simulink model "Practica1MSF "  (R2025b)
settings: Solver=VariableStepAuto  StartTime=0.0  StopTime=10  MaxStep=1E-3  RelTol=1e-3
libraries: slpidlib x1, simulink x1
settings DataIOCC: ReturnWorkspaceOutputs=off  TimeSaveName=t
settings DebuggingCC: AlgebraicLoopMsg=none  ArtificialAlgebraicLoopMsg=none  MaxConsecutiveZCsMsg=none

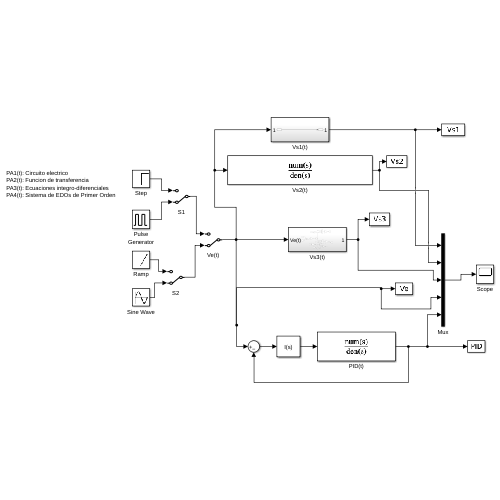
[thumbnail: Simulink's stored preview of the top-level diagram]
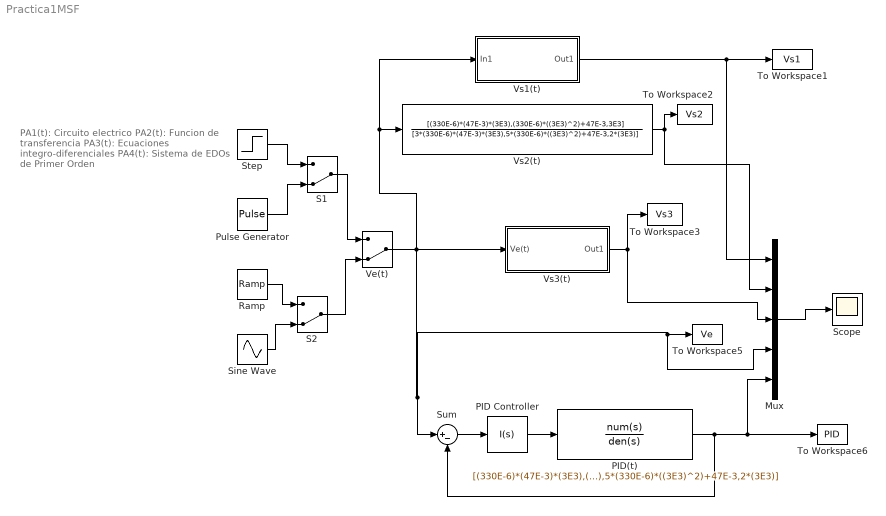
== system Practica1MSF  ==
  note: PA1(t): Circuito electrico
      | PA2(t): Funcion de transferencia
      | PA3(t): Ecuaciones integro-diferenciales
      | PA4(t): Sistema de EDOs de Primer Orden
  Mux : Mux  Inputs=5
  PID Controller : slpidlib/PID Controller  Controller=I  Form=Parallel  TimeDomain=Continuous-time  UseExternalTs=off  SampleTime=-1  IntegratorMethod=Forward Euler  FilterMethod=Forward Euler  ControllerParametersSource=internal  P=1  I=1961.8958  UseKiTs=off  D=1  UseExternalDerivativeSource=off  N=1  UseFilter=on  TunerSelectOption=Transfer Function Based (PID Tuner App)  InitialConditionSource=internal  InitialConditionForIntegrator=0  InitialConditionForFilter=0  DifferentiatorICPrevScaledInput=0  ExternalReset=none  TrackingMode=off  Kt=1  LimitOutput=off  SatLimitsSource=internal  UpperSaturationLimit=inf  LowerSaturationLimit=-inf  LinearizeAsGain=on  AntiWindupMode=none  Kb=1  LimitIntegrator=off  UpperIntegratorSaturationLimit=inf  LowerIntegratorSaturationLimit=-inf  POutMin=[]  POutMax=[]  IOutMin=[]  IOutMax=[]  DOutMin=[]  DOutMax=[]  NOutMin=[]  NOutMax=[]  SumOutMin=[]  SumOutMax=[]  SaturationOutMin=[]  SaturationOutMax=[]  PParamMin=[]  PParamMax=[]  IParamMin=[]  IParamMax=[]  DParamMin=[]  DParamMax=[]  NParamMin=[]  NParamMax=[]  KbParamMin=[]  KbParamMax=[]  KtParamMin=[]  KtParamMax=[]  KbOutMin=[]  KbOutMax=[]  KtOutMin=[]  KtOutMax=[]  IntegratorOutMin=[]  IntegratorOutMax=[]  FilterOutMin=[]  FilterOutMax=[]  SumI1OutMin=[]  SumI1OutMax=[]  SumI2OutMin=[]  SumI2OutMax=[]  SumI3OutMin=[]  SumI3OutMax=[]  SumI4OutMin=[]  SumI4OutMax=[]  SumDOutMin=[]  SumDOutMax=[]  DifferentiatorOutMin=[]  DifferentiatorOutMax=[]  FilterDiffOutCoefMin=[]  FilterDiffOutCoefMax=[]  ReciprocalOutMin=[]  ReciprocalOutMax=[]  SumDenOutMin=[]  SumDenOutMax=[]  SumNumOutMin=[]  SumNumOutMax=[]  DivideOutMin=[]  DivideOutMax=[]  UdiffTsProdOutMin=[]  UdiffTsProdOutMax=[]  NTsProdOutMin=[]  NTsProdOutMax=[]  UintegralTsProdOutMin=[]  UintegralTsProdOutMax=[]  UngainTsProdOutMin=[]  UngainTsProdOutMax=[]  ClampingZeroOutDataTypeStr=Inherit: Inherit via back propagation  ClampingZeroOutMin=[]  ClampingZeroOutMax=[]  FilterDenConstantOutDataTypeStr=Inherit: Inherit via back propagation  FilterDenConstantOutMin=[]  FilterDenConstantOutMax=[]  PCopyOutDataTypeStr=Inherit: Inherit via back propagation  PCopyOutMin=[]  PCopyOutMax=[]  NCopyOutDataTypeStr=Inherit: Inherit via back propagation  NCopyOutMin=[]  NCopyOutMax=[]  IntegratorContinuousStateAttributes=''  IntegratorStateMustResolveToSignalObject=off  IntegratorRTWStateStorageClass=Auto  FilterContinuousStateAttributes=''  FilterStateMustResolveToSignalObject=off  FilterRTWStateStorageClass=Auto  ParallelPVariant=Disabled  IdealPVariant=Disabled  IVariant=InternalParameters  DVariant=Disabled  IntegratorVariant=Continuous  SatVariant=Disabled  AWVariant=Passthrough  PCopyVariant=Disabled  TRVariant=Disabled  FdbkBlocksVariant=Forward  IdealPFdbkVariant=Disabled  SatFdbkVariant=Disabled  DerivativeFilterVariant=Disabled  NVariant=Disabled  NCopyVariant=Disabled_SignalSpec  FilterICVariant=Disabled  IntegratorICVariant=InternalICs  ExternalResetVariant=Disabled  TRSumVariant=Passthrough  SumFdbkVariant=Disabled  SumVariant=Passthrough_I  TsampFilterVariant=InternalTs  TsampNgainVariant=Passthrough  TsampIntegralVariant=Disabled_SignalSpec  ExternalSaturationOutDataTypeStr=Inherit: Same as second input  DerivativeSourceVariant=Disabled  PreIntVariant=InternalPreInt
  PID(t) : TransferFcn  Numerator=[(330E-6)*(47E-3)*(3E3),(330E-6)*((3E3)^2)+47E-3,3E3]  Denominator=[3*(330E-6)*(47E-3)*(3E3),5*(330E-6)*((3E3)^2)+47E-3,2*(3E3)]
  Pulse Generator : DiscretePulseGenerator  PulseType=Time based  Period=10  PulseWidth=10  PhaseDelay=1
  Ramp : simulink/Sources/Ramp  slope=1/10  start=0  InitialOutput=0
  S1 : ManualSwitch  CurrentSetting=0
  S2 : ManualSwitch  CurrentSetting=0
  Scope : Scope
      settings: ActiveDisplayYMinimum=-0.12518759179665592  ActiveDisplayYMaximum=1.1266883261699037
  Sine Wave : Sin  Frequency=pi/2  SampleTime=0
  Step : Step  Time=0  Before=1  SampleTime=0
  Sum : Sum  Inputs=|+-
  To Workspace1 : ToWorkspace  VariableName=Vs1  SampleTime=-1
  To Workspace2 : ToWorkspace  VariableName=Vs2  SampleTime=-1
  To Workspace3 : ToWorkspace  VariableName=Vs3  SampleTime=-1
  To Workspace5 : ToWorkspace  VariableName=Ve  SampleTime=-1
  To Workspace6 : ToWorkspace  VariableName=PID  SampleTime=-1
  Ve(t) : ManualSwitch  CurrentSetting=0
  Vs1(t) : Subsystem
  Vs2(t) : TransferFcn  Numerator=[(330E-6)*(47E-3)*(3E3),(330E-6)*((3E3)^2)+47E-3,3E3]  Denominator=[3*(330E-6)*(47E-3)*(3E3),5*(330E-6)*((3E3)^2)+47E-3,2*(3E3)]
  Vs3(t) : Subsystem
  wires:
  Step/1 -> S1/1
  Pulse Generator/1 -> S1/2
  Ramp/1 -> S2/1
  Sine Wave/1 -> S2/2
  S1/1 -> Ve(t)/1
  S2/1 -> Ve(t)/2
  Vs2(t)/1 -> To Workspace2/1, Mux/2
  Ve(t)/1 -> Vs3(t)/1(Ve(t)), Vs2(t)/1, Vs1(t)/1(In1), Sum/1, Mux/4, To Workspace5/1
  Mux/1 -> Scope/1
  Vs1(t)/1(Out1) -> To Workspace1/1, Mux/1
  PID Controller/1 -> PID(t)/1
  Sum/1 -> PID Controller/1
  Vs3(t)/1(Out1) -> To Workspace3/1, Mux/3
  PID(t)/1 -> Sum/2, Mux/5, To Workspace6/1

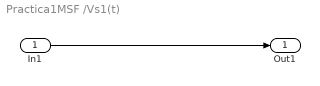
== system Practica1MSF /Vs1(t) ==
  In1 : Inport
  Out1 : Outport
  wires:
  In1/1 -> Out1/1

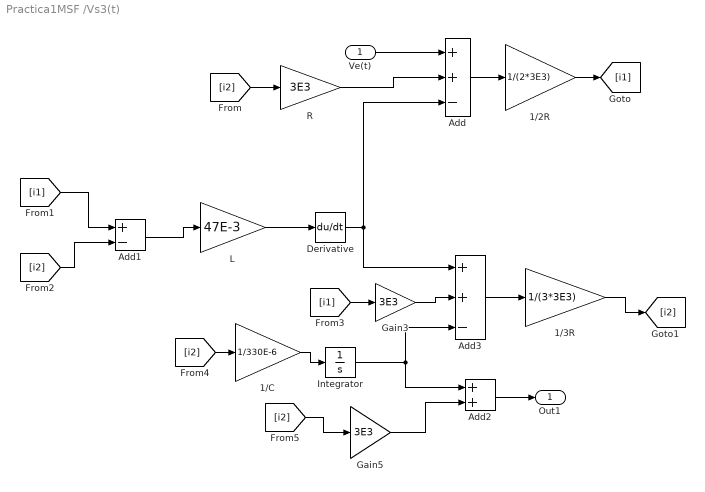
== system Practica1MSF /Vs3(t) ==
  Ve(t) : Inport
  1/2R : Gain  Gain=1/(2*3E3)
  1/3R : Gain  Gain=1/(3*3E3)
  1/C : Gain  Gain=1/330E-6
  Add : Sum  Inputs=++-
  Add1 : Sum  Inputs=+-
  Add2 : Sum
  Add3 : Sum  Inputs=++-
  Derivative : Derivative
  Gain3 : Gain  Gain=3E3
  Gain5 : Gain  Gain=3E3
  Integrator : Integrator
  L : Gain  Gain=47E-3
  R : Gain  Gain=3E3
  Out1 : Outport
  wires:
  Ve(t)/1 -> Add/1
  [i2] -> R/1
  R/1 -> Add/2
  Add/1 -> 1/2R/1
  1/2R/1 -> [i1]
  [i1] -> Add1/1
  [i2] -> Add1/2
  Add1/1 -> L/1
  L/1 -> Derivative/1
  Derivative/1 -> Add3/1, Add/3
  [i1] -> Gain3/1
  Gain3/1 -> Add3/2
  [i2] -> 1/C/1
  1/C/1 -> Integrator/1
  Integrator/1 -> Add2/1, Add3/3
  Add2/1 -> Out1/1
  [i2] -> Gain5/1
  Gain5/1 -> Add2/2
  Add3/1 -> 1/3R/1
  1/3R/1 -> [i2]
